simulink model "Lab1"  (R2021a)
settings: Solver=VariableStepAuto  StartTime=0.0  StopTime=500  RelTol=1e-3
values from neighbouring files (symbols this model uses):
  c0 = 2.35    [Laboratory1.m]
  ci = evalin('base','ci')    [Laboratory1.m]
  Edr = evalin('base','Edr')    [Laboratory1.m]
  hA = evalin('base','hA')    [Laboratory1.m]
  k0 = evalin('base','k0')    [Laboratory1.m]
  minusdeltaH = 24953    [Laboratory1.m]
  q = evalin('base','q')    [Laboratory1.m]
  rcp = evalin('base','rcp')    [Laboratory1.m]
  T0 = 368    [Laboratory1.m]
  Ti = evalin('base','Ti')    [Laboratory1.m]
  Tr = evalin('base','Tr')    [Laboratory1.m]
  V = evalin('base','V')    [Laboratory1.m]
settings Model: Creator=Automatica  LastModifiedBy=Automatica

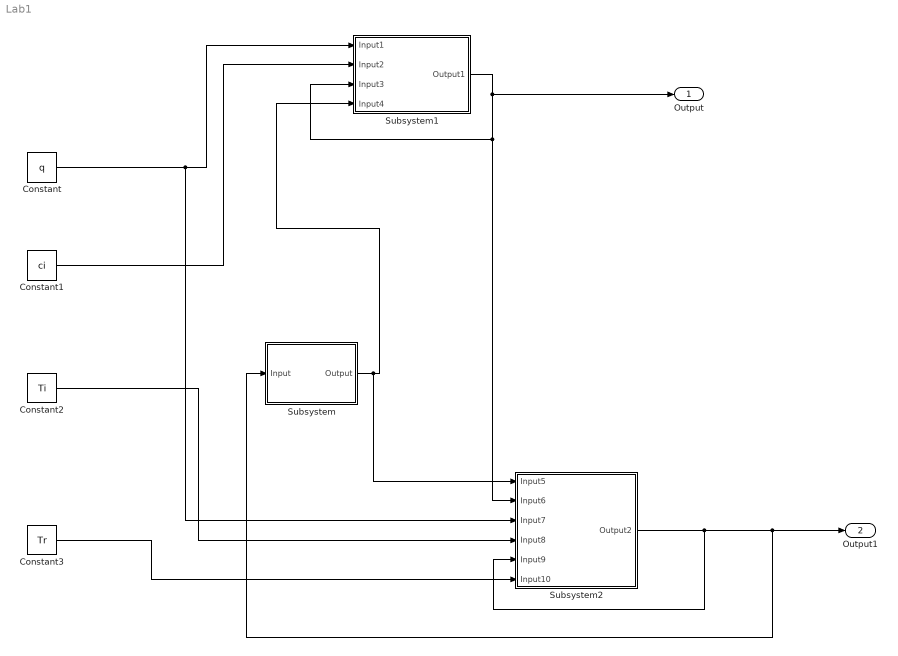
== system Lab1 ==
  Constant : Constant  Value=q
  Constant1 : Constant  Value=ci
  Constant2 : Constant  Value=Ti
  Constant3 : Constant  Value=Tr
  Subsystem : Subsystem
  Subsystem1 : Subsystem
  Subsystem2 : Subsystem
  Output : Outport
  Output1 : Outport  Port=2
  wires:
  Constant/1 -> Subsystem2/3(Input7), Subsystem1/1(Input1)
  Constant1/1 -> Subsystem1/2(Input2)
  Subsystem/1(Output) -> Subsystem2/1(Input5), Subsystem1/4(Input4)
  Subsystem1/1(Output1) -> Subsystem2/2(Input6), Subsystem1/3(Input3), Output/1
  Subsystem2/1(Output2) -> Subsystem2/5(Input9), Subsystem/1(Input), Output1/1
  Constant3/1 -> Subsystem2/6(Input10)
  Constant2/1 -> Subsystem2/4(Input8)

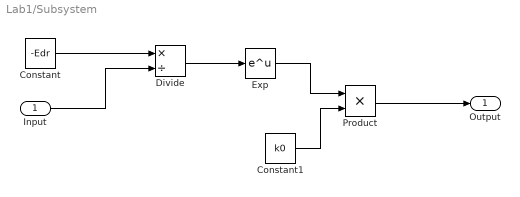
== system Lab1/Subsystem ==
  Input : Inport
  Constant : Constant  Value=-Edr
  Constant1 : Constant  Value=k0
  Divide : Product  Inputs=*/
  Exp : Math  SaturateOnIntegerOverflow=on
  Product : Product
  Output : Outport
  wires:
  Exp/1 -> Product/1
  Constant/1 -> Divide/1
  Product/1 -> Output/1
  Divide/1 -> Exp/1
  Constant1/1 -> Product/2
  Input/1 -> Divide/2

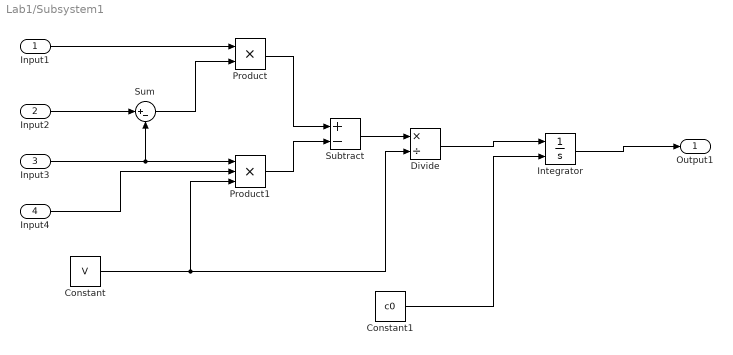
== system Lab1/Subsystem1 ==
  Input1 : Inport
  Input2 : Inport  Port=2
  Input3 : Inport  Port=3
  Input4 : Inport  Port=4
  Constant : Constant  Value=V
  Constant1 : Constant  Value=c0
  Divide : Product  Inputs=*/
  Integrator : Integrator  InitialConditionSource=external  InitialCondition=c0
  Product : Product
  Product1 : Product  Inputs=3
  Subtract : Sum  Inputs=+-
  Sum : Sum  Inputs=|+-
  Output1 : Outport
  wires:
  Product/1 -> Subtract/1
  Integrator/1 -> Output1/1
  Divide/1 -> Integrator/1
  Subtract/1 -> Divide/1
  Input1/1 -> Product/1
  Constant/1 -> Divide/2, Product1/3
  Sum/1 -> Product/2
  Constant1/1 -> Integrator/2
  Input3/1 -> Sum/2, Product1/1
  Input2/1 -> Sum/1
  Input4/1 -> Product1/2
  Product1/1 -> Subtract/2

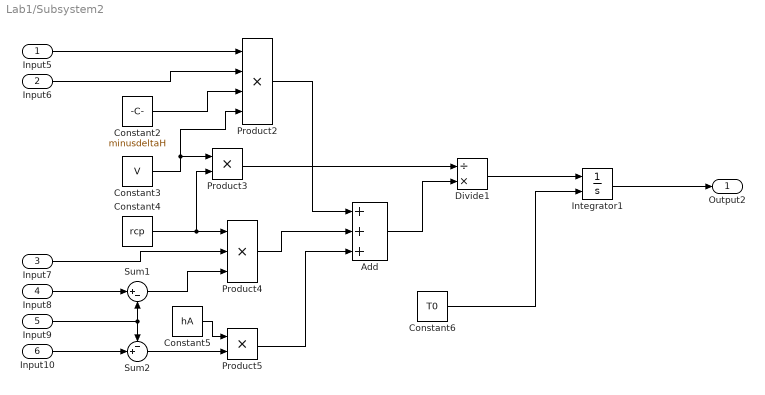
== system Lab1/Subsystem2 ==
  Input5 : Inport
  Input6 : Inport  Port=2
  Input7 : Inport  Port=3
  Input8 : Inport  Port=4
  Input9 : Inport  Port=5
  Input10 : Inport  Port=6
  Add : Sum  Inputs=+++
  Constant2 : Constant  Value=minusdeltaH
  Constant3 : Constant  Value=V
  Constant4 : Constant  Value=rcp
  Constant5 : Constant  Value=hA
  Constant6 : Constant  Value=T0
  Divide1 : Product  Inputs=/*
  Integrator1 : Integrator  InitialConditionSource=external  InitialCondition=c0
  Product2 : Product  Inputs=4
  Product3 : Product
  Product4 : Product  Inputs=3
  Product5 : Product
  Sum1 : Sum  Inputs=|+-
  Sum2 : Sum  Inputs=-+|
  Output2 : Outport
  wires:
  Constant4/1 -> Product4/1, Product3/2
  Add/1 -> Divide1/2
  Input9/1 -> Sum2/1, Sum1/2
  Input10/1 -> Sum2/2
  Sum2/1 -> Product5/2
  Divide1/1 -> Integrator1/1
  Constant2/1 -> Product2/3
  Constant3/1 -> Product3/1, Product2/4
  Product5/1 -> Add/3
  Constant6/1 -> Integrator1/2
  Product3/1 -> Divide1/1
  Product4/1 -> Add/2
  Input5/1 -> Product2/1
  Input6/1 -> Product2/2
  Product2/1 -> Add/1
  Input8/1 -> Sum1/1
  Sum1/1 -> Product4/3
  Integrator1/1 -> Output2/1
  Constant5/1 -> Product5/1
  Input7/1 -> Product4/2
